simulink model "slo_distpipe_lut"  (R2015b)
settings: Solver=FixedStepDiscrete  SolverMode=SingleTasking  StartTime=0.0  StopTime=10.0  RelTol=1e-3
libraries: simulink x4
settings Model: Creator=amatsumo  LastModifiedBy=amatsumo
settings DataIOCC: SaveFormat=Array  SignalLoggingSaveFormat=ModelDataLogs  SaveOutput=off  SignalLogging=off  SaveTime=off
settings OptimizationCC: BlockReduction=off  ConditionallyExecuteInputs=off  DefaultParameterBehavior=Inlined  ExpressionDepthLimit=2147483647
settings DebuggingCC: AlgebraicLoopMsg=error  UnderspecifiedInitializationDetection=Classic  MergeDetectMultiDrivingBlocksExec=none  SolverPrmCheckMsg=warning  InheritedTsInSrcMsg=none  SingleTaskRateTransMsg=error  FcnCallInpInsideContextMsg=UseLocalSettings  StateNameClashWarn=warning
settings HardwareCC: ProdBitPerPointer=32  ProdLargestAtomicFloat=None  ProdIntDivRoundTo=Undefined  ProdEndianess=Unspecified  ProdWordSize=32  ProdHWDeviceType=ASIC/FPGA->ASIC/FPGA  ProdEqTarget=off
settings GRTTargetCC: GeneratePreprocessorConditionals=Disable all  CombineOutputUpdateFcns=off  GRTInterface=on
settings ConfigComp: CovModelRefEnable=Off  CovSFcnEnable=off

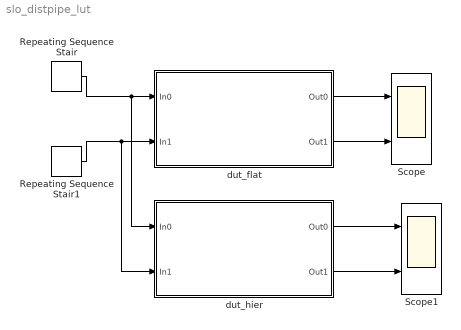
== system slo_distpipe_lut ==
  Repeating Sequence Stair : simulink/Sources/Repeating Sequence Stair  OutValues=[1 2 3].'  tsamp=1  OutMin=[]  OutMax=[]  OutDataTypeStr=fixdt(1,8,0)  OutputDataTypeScalingMode=Specify via dialog  OutDataType=fixdt(1,8,0)  ConRadixGroup=Best Precision: Vector-wise  OutScaling=[]
  Repeating Sequence Stair1 : simulink/Sources/Repeating Sequence Stair  OutValues=[1 3 4 5].'  tsamp=1  OutMin=[]  OutMax=[]  OutDataTypeStr=uint8  OutputDataTypeScalingMode=uint8  OutDataType=fixdt(1,8,0)  ConRadixGroup=Best Precision: Vector-wise  OutScaling=[]
  Scope : Scope  NumInputPorts=2
  Scope1 : Scope  NumInputPorts=2
  dut_flat : Subsystem
  dut_hier : Subsystem
  wires:
  dut_flat/1(Out0) -> Scope/1
  Repeating Sequence Stair/1 -> dut_hier/1(In0), dut_flat/1(In0)
  Repeating Sequence Stair1/1 -> dut_hier/2(In1), dut_flat/2(In1)
  dut_flat/2(Out1) -> Scope/2
  dut_hier/1(Out0) -> Scope1/1
  dut_hier/2(Out1) -> Scope1/2

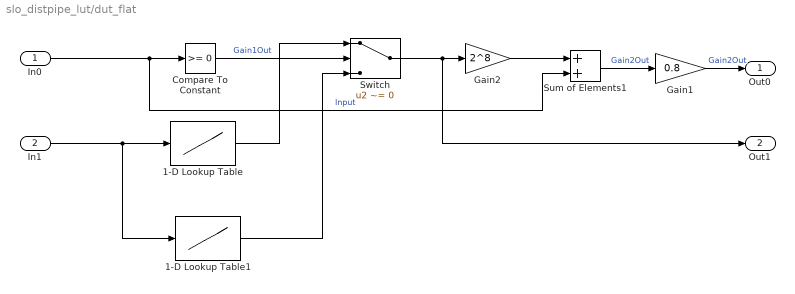
== system slo_distpipe_lut/dut_flat ==
  In0 : Inport
  In1 : Inport  Port=2
  1-D Lookup Table : Lookup_n-D  NumberOfTableDimensions=1  BreakpointsForDimension1=[0:255]  IndexSearchMethod=Evenly spaced points  Table=atan(([0:255]-128)/128*5)  InterpMethod=Flat  DiagnosticForOutOfRangeInput=Error  OutDataTypeStr=fixdt(1,16,14)  RndMeth=Zero  InputSameDT=on
  1-D Lookup Table1 : Lookup_n-D  NumberOfTableDimensions=1  BreakpointsForDimension1=[0:255]  IndexSearchMethod=Evenly spaced points  Table=tanh(([0:255]-128)/128*5)  InterpMethod=Flat  DiagnosticForOutOfRangeInput=Error  OutDataTypeStr=fixdt(1,16,14)  RndMeth=Zero  InputSameDT=on
  Compare To Constant : simulink/Logic and Bit Operations/Compare To Constant  relop=>=  const=0  OutDataTypeStr=boolean
  Gain1 : Gain  Gain=0.8  RndMeth=Nearest  OutDataTypeStr=Inherit: Same as input
  Gain2 : Gain  Gain=2^8  OutDataTypeStr=fixdt(1,16,6)  RndMeth=Nearest
  Sum of Elements1 : Sum  OutDataTypeStr=Inherit: Same as first input
  Switch : Switch  Criteria=u2 ~= 0
  Out0 : Outport
  Out1 : Outport  Port=2
  wires:
  Switch/1 -> Gain2/1, Out1/1
  In1/1 -> 1-D Lookup Table1/1, 1-D Lookup Table/1
  In0/1 -> Sum of Elements1/2, Compare To Constant/1  "Input"
  Sum of Elements1/1 -> Gain1/1  "Gain2Out"
  Gain1/1 -> Out0/1  "Gain2Out"
  1-D Lookup Table1/1 -> Switch/3
  1-D Lookup Table/1 -> Switch/1
  Compare To Constant/1 -> Switch/2  "Gain1Out"
  Gain2/1 -> Sum of Elements1/1

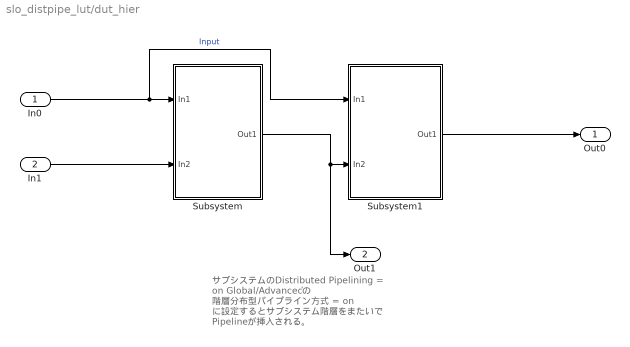
== system slo_distpipe_lut/dut_hier ==
  note: サブシステムのDistributed Pipelining = on
      | Global/Advancedの
      | 階層分布型パイプライン方式 = on
      | に設定するとサブシステム階層をまたいで
      | Pipelineが挿入される。
  In0 : Inport
  In1 : Inport  Port=2
  Subsystem : Subsystem
  Subsystem1 : Subsystem
  Out0 : Outport
  Out1 : Outport  Port=2
  wires:
  In0/1 -> Subsystem1/1(In1), Subsystem/1(In1)  "Input"
  Subsystem/1(Out1) -> Out1/1, Subsystem1/2(In2)
  In1/1 -> Subsystem/2(In2)
  Subsystem1/1(Out1) -> Out0/1

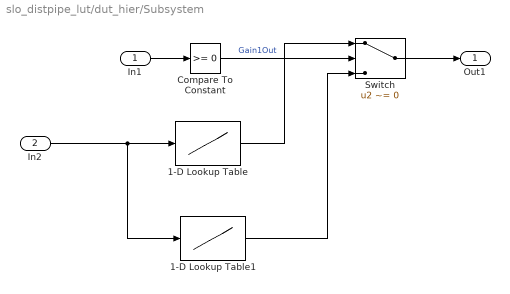
== system slo_distpipe_lut/dut_hier/Subsystem ==
  In1 : Inport
  In2 : Inport  Port=2
  1-D Lookup Table : Lookup_n-D  NumberOfTableDimensions=1  BreakpointsForDimension1=[0:255]  IndexSearchMethod=Evenly spaced points  Table=atan(([0:255]-128)/128*5)  InterpMethod=Flat  DiagnosticForOutOfRangeInput=Error  OutDataTypeStr=fixdt(1,16,14)  RndMeth=Zero  InputSameDT=on
  1-D Lookup Table1 : Lookup_n-D  NumberOfTableDimensions=1  BreakpointsForDimension1=[0:255]  IndexSearchMethod=Evenly spaced points  Table=tanh(([0:255]-128)/128*5)  InterpMethod=Flat  DiagnosticForOutOfRangeInput=Error  OutDataTypeStr=fixdt(1,16,14)  RndMeth=Zero  InputSameDT=on
  Compare To Constant : simulink/Logic and Bit Operations/Compare To Constant  relop=>=  const=0  OutDataTypeStr=boolean
  Switch : Switch  Criteria=u2 ~= 0
  Out1 : Outport
  wires:
  Compare To Constant/1 -> Switch/2  "Gain1Out"
  1-D Lookup Table/1 -> Switch/1
  In1/1 -> Compare To Constant/1
  Switch/1 -> Out1/1
  In2/1 -> 1-D Lookup Table/1, 1-D Lookup Table1/1
  1-D Lookup Table1/1 -> Switch/3

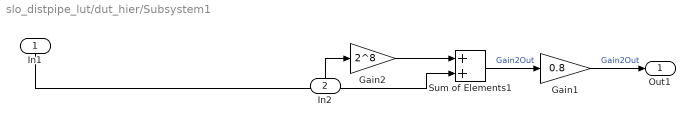
== system slo_distpipe_lut/dut_hier/Subsystem1 ==
  In1 : Inport
  In2 : Inport  Port=2
  Gain1 : Gain  Gain=0.8  RndMeth=Nearest  OutDataTypeStr=Inherit: Same as input
  Gain2 : Gain  Gain=2^8  OutDataTypeStr=fixdt(1,16,6)  RndMeth=Nearest
  Sum of Elements1 : Sum  OutDataTypeStr=Inherit: Same as first input
  Out1 : Outport
  wires:
  In1/1 -> Sum of Elements1/2
  Gain1/1 -> Out1/1  "Gain2Out"
  Gain2/1 -> Sum of Elements1/1
  In2/1 -> Gain2/1
  Sum of Elements1/1 -> Gain1/1  "Gain2Out"
